simulink model "regulacion_nominal_modelo_lineal"  (R2021a)
settings: Solver=VariableStepAuto  StartTime=0.0  StopTime=300  RelTol=1e-3
settings Model: Creator=jmata  LastModifiedBy=jmata

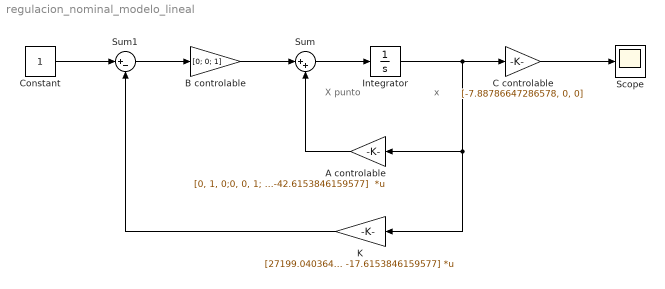
== system regulacion_nominal_modelo_lineal ==
  note: x
  note: X punto
  A controlable : Gain  Gain=[0, 1, 0;0, 0, 1; 26809.0403648094 , 629.09300494194, -42.6153846159577]  Multiplication=Matrix(K*u)
  B controlable : Gain  Gain=[0; 0; 1]
  C controlable : Gain  Gain=[-7.88786647286578, 0, 0]
  Constant : Constant
  Integrator : Integrator
  K : Gain  Gain=[27199.0403648094, 805.093004941941, -17.6153846159577]  Multiplication=Matrix(K*u)
  Scope : Scope
  Sum : Sum  Inputs=|++
  Sum1 : Sum  Inputs=|+-
  wires:
  A controlable/1 -> Sum/2
  B controlable/1 -> Sum/1
  Sum/1 -> Integrator/1
  Integrator/1 -> K/1, A controlable/1, C controlable/1
  C controlable/1 -> Scope/1
  Constant/1 -> Sum1/1
  Sum1/1 -> B controlable/1
  K/1 -> Sum1/2
